simulink model "CCS_2"  (R2019b)
settings: Solver=FixedStepAuto  StartTime=0.0  StopTime=5.0  FixedStep=0.1  RelTol=1e-3
libraries: simulink x1
settings Model: Creator=Administrator  LastModifiedBy=Administrator

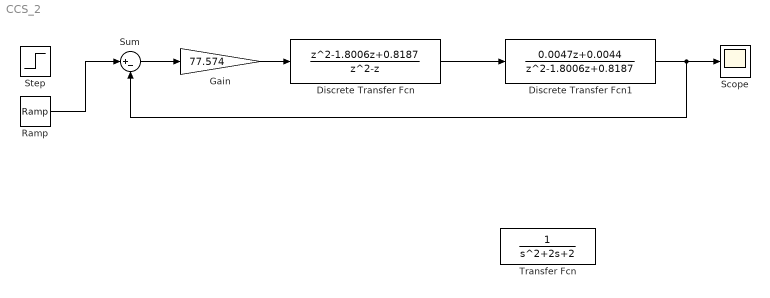
== system CCS_2 ==
  Discrete Transfer Fcn : DiscreteTransferFcn  Numerator=[1 -1.8006 0.8187]  Denominator=[1 -1 0]
  Discrete Transfer Fcn1 : DiscreteTransferFcn  Numerator=[0.0047 0.0044]  Denominator=[1 -1.8006 0.8187]
  Gain : Gain  Gain=77.574
  Ramp : simulink/Sources/Ramp  slope=1  start=0  InitialOutput=0
  Scope : Scope
  Step : Step  Time=0  SampleTime=0
  Sum : Sum  Inputs=|+-
  Transfer Fcn : TransferFcn  Denominator=[1 2 2]
  wires:
  Sum/1 -> Gain/1
  Gain/1 -> Discrete Transfer Fcn/1
  Discrete Transfer Fcn1/1 -> Sum/2, Scope/1
  Discrete Transfer Fcn/1 -> Discrete Transfer Fcn1/1
  Ramp/1 -> Sum/1
